simulink model "qd2ab"  (R2021a)
settings: Solver=VariableStepAuto  StartTime=0.0  StopTime=10.0  RelTol=1e-3
settings Model: Creator=Utkarsh Anand  LastModifiedBy=Utkarsh Anand
settings DataIOCC: SaveOutput=off  SaveTime=off

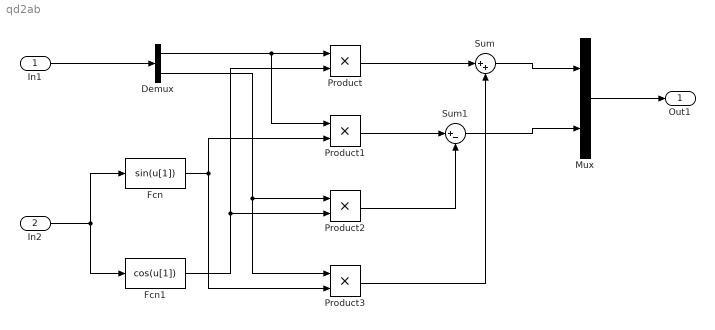
== system qd2ab ==
  In1 : Inport  OutDataTypeStr=double  PortDimensions=2  SampleTime=0
  In2 : Inport  Port=2  OutDataTypeStr=double  PortDimensions=1  SampleTime=0
  Demux : Demux  Outputs=2
  Fcn : Fcn
  Fcn1 : Fcn  Expr=cos(u[1])
  Mux : Mux  Inputs=2
  Product{,1..3} (4 alike) : Product
  Sum : Sum  Inputs=|++
  Sum1 : Sum  Inputs=|+-
  Out1 : Outport  OutDataTypeStr=double  PortDimensions=2  SampleTime=0
  wires:
  Sum1/1 -> Mux/2
  Demux/1 -> Product/1, Product1/1
  Fcn1/1 -> Product/2, Product2/2
  Sum/1 -> Mux/1
  Product/1 -> Sum/1
  Demux/2 -> Product2/1, Product3/1
  In2/1 -> Fcn1/1, Fcn/1
  Product2/1 -> Sum1/2
  Fcn/1 -> Product3/2, Product1/2
  Mux/1 -> Out1/1
  Product1/1 -> Sum1/1
  Product3/1 -> Sum/2
  In1/1 -> Demux/1
